simulink model "bridge1"  (R2020b)
settings: Solver=VariableStepAuto  StartTime=0.0  StopTime=10.0  RelTol=1e-3
libraries: fl_lib x6, nesl_utility x1, ee_lib x1
settings Model: Creator=Miodrag Bolic  LastModifiedBy=bolic

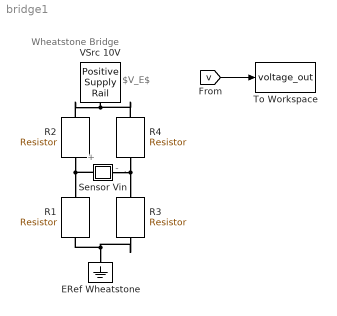
== system bridge1 ==
  note: -
  note: +
  note: Wheatstone
      | Bridge
  note: $V_E$
  ERef Wheatstone : fl_lib/Electrical/Electrical Elements/Electrical Reference
      settings: SourceProductName=Foundation Library
  R{1..4} (4 alike) : fl_lib/Electrical/Electrical Elements/Resistor  R=120 Ohm  i_specify=off  i_priority=High  i=0 A  i_nominal_specify=off  i_nominal_unit=A  i_nominal_value=1  v_specify=off  v_priority=High  v=0 V  v_nominal_specify=off  v_nominal_unit=V  v_nominal_value=1
      settings: SourceProductName=Foundation Library
  Sensor Vin : Subsystem
      mask Display: disp('Vo')
  To Workspace : ToWorkspace  VariableName=voltage_out  SaveFormat=Timeseries  SampleTime=-1
  VSrc 10V : ee_lib/Sources/Positive Supply Rail  v0=5 V
      settings: SourceProductName=Electrical  InternalSimscapePortConfiguration="{\"Bottom\":[],\"Left\":[],\"Right\":[{\"id\":\"p\",\"label\":\"\",\"type\":\"foundation.electrical.electrical\"}],\"Top\":[]}"
  wires:
  [v] -> To Workspace/1
  connections:
  R4/LConn1 -- R2/LConn1 -- VSrc 10V/RConn1
  R4/RConn1 -- Sensor Vin/RConn1 -- R3/LConn1
  R2/RConn1 -- R1/LConn1 -- Sensor Vin/LConn1
  ERef Wheatstone/LConn1 -- R3/RConn1 -- R1/RConn1

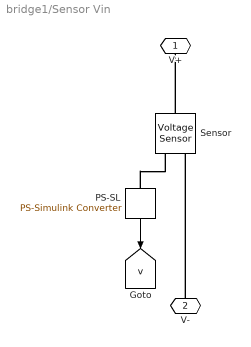
== system bridge1/Sensor Vin ==
  PS-SL : nesl_utility/PS-Simulink Converter  PhysicalDomain=network_engine_domain  SubClassName=ps_output  LeftPortType=input  RightPortType=output  PseudoPeriodic=off  Frequencies=[]  Unit=1  AffineConversion=off
  Sensor : fl_lib/Electrical/Electrical Sensors/Voltage Sensor
      settings: SourceProductName=Foundation Library
  V+ : PMIOPort  Side=Right
  V- : PMIOPort  Port=2  Side=Left
  tag scope: v=global
  wires:
  PS-SL/1 -> [v]
  connections:
  PS-SL/LConn1 -- Sensor/RConn1
  Sensor/LConn1 -- V+/RConn1
  V-/RConn1 -- Sensor/RConn2
